simulink model "pipelined_adc"  (R2019a)
settings: Solver=FixedStepDiscrete  StartTime=0.0  StopTime=30000  FixedStep=1  RelTol=1e-3
libraries: pipelined_adc_library x5
settings Model: Creator=johan  LastModifiedBy=johan

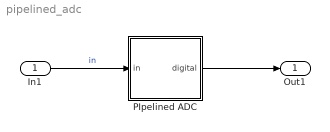
== system pipelined_adc ==
  In1 : Inport
  PIpelined ADC : Subsystem
  Out1 : Outport
  wires:
  PIpelined ADC/1(digital) -> Out1/1
  In1/1 -> PIpelined ADC/1(in)  "in"

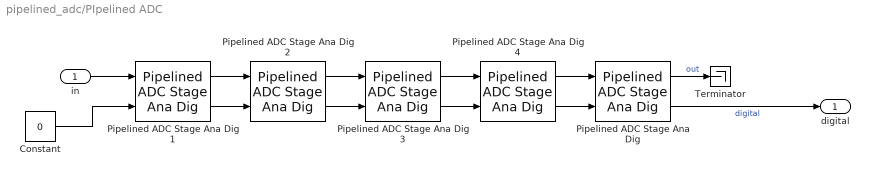
== system pipelined_adc/PIpelined ADC ==
  in : Inport
  Constant : Constant  Value=0
  Pipelined ADC Stage Ana Dig : pipelined_adc_library/Pipelined ADC Stage Ana Dig  comp_offsets=[0, 0, 0, 0, 0, 0]  sigma_noise=1e-3/16  delta_G=0
  Pipelined ADC Stage Ana Dig 1 : pipelined_adc_library/Pipelined ADC Stage Ana Dig  comp_offsets=[0, 0, 0, 0, 0, 0]  sigma_noise=1e-3  delta_G=3e-3
  Pipelined ADC Stage Ana Dig 2 : pipelined_adc_library/Pipelined ADC Stage Ana Dig  comp_offsets=[0, 0, 0, 0, 0, 0]  sigma_noise=1e-3/2  delta_G=0
  Pipelined ADC Stage Ana Dig 3 : pipelined_adc_library/Pipelined ADC Stage Ana Dig  comp_offsets=[0, 0, 0, 0, 0, 0]  sigma_noise=1e-3/4  delta_G=0
  Pipelined ADC Stage Ana Dig 4 : pipelined_adc_library/Pipelined ADC Stage Ana Dig  comp_offsets=[0, 0, 0, 0, 0, 0]  sigma_noise=1e-3/8  delta_G=0
  Terminator : Terminator
  digital : Outport
  wires:
  Pipelined ADC Stage Ana Dig 2/1 -> Pipelined ADC Stage Ana Dig 3/1
  Constant/1 -> Pipelined ADC Stage Ana Dig 1/2
  Pipelined ADC Stage Ana Dig/1 -> Terminator/1  "out"
  Pipelined ADC Stage Ana Dig 1/1 -> Pipelined ADC Stage Ana Dig 2/1
  Pipelined ADC Stage Ana Dig 4/1 -> Pipelined ADC Stage Ana Dig/1
  Pipelined ADC Stage Ana Dig 2/2 -> Pipelined ADC Stage Ana Dig 3/2
  Pipelined ADC Stage Ana Dig 3/2 -> Pipelined ADC Stage Ana Dig 4/2
  Pipelined ADC Stage Ana Dig 1/2 -> Pipelined ADC Stage Ana Dig 2/2
  Pipelined ADC Stage Ana Dig/2 -> digital/1  "digital"
  Pipelined ADC Stage Ana Dig 3/1 -> Pipelined ADC Stage Ana Dig 4/1
  Pipelined ADC Stage Ana Dig 4/2 -> Pipelined ADC Stage Ana Dig/2
  in/1 -> Pipelined ADC Stage Ana Dig 1/1
